simulink model "GCI_Ctrl_PLL_C2000"  (R2024a)
settings: Solver=FixedStepDiscrete  StartTime=0.0  StopTime=8  FixedStep=Sim.ContSampleTime  RelTol=1e-3  EnableMultiTasking=on
values from neighbouring files (symbols this model uses):
  ADPTV = 1.3912    [ModelDD.sldd]
  Ctrl = 0    [ModelDD.sldd]
  EnableMonitors = 0    [ModelDD.sldd]
  FrcPwr = 1    [ModelDD.sldd]
  IdSp = 0.0    [ModelDD.sldd]
  IqSp = 0.0    [ModelDD.sldd]
  ModReq = 1    [ModelDD.sldd]
  PorISel = 0    [ModelDD.sldd]
  PSp = 0.0    [ModelDD.sldd]
  QSp = 0.0    [ModelDD.sldd]
  Sim : value not decoded    [ModelDD.sldd]
  Test = 0    [ModelDD.sldd]
  Var = 650.0    [ModelDD.sldd]
undefined symbols (not defined in the file or in its folder): DiscIntNeverNeededParam, Down, GPTRIP1SEL, GPTRIP2SEL, magnitude, P, TZ1, TZ2, Up
libraries: simulink x38, c2837xDlib x22, c2802xlib x15, slpidlib x9, spsMeanLib x9, spsCurrentMeasurementLib x7, spsThreePhaseVIMeasurementLib x5, spsVoltageMeasurementLib x5, spsTHDLib x4, spsSeriesRLCBranchLib x4, svdutilitieslib x3, c280xlib x3
(part 7 of 11)

== system GCI_Ctrl_PLL_C2000/C2000_SW/CtrlLoop/PLL_Vref/Subsystem/LPF2 ==
  u : Inport
  Alpha : Gain  Gain=(2-w*Ts)/(2+w*Ts)
  Beta : Gain  Gain=(w*Ts)/(2+w*Ts)
  Delay1 : Delay  DelayLength=1  InitialCondition=y_0
  Delay2 : Delay  DelayLength=1
  Sum1 : Sum  Inputs=++|
  Sum2 : Sum  Inputs=|++
  y : Outport  VectorParamsAs1DForOutWhenUnconnected=off
  wires:
  Sum2/1 -> y/1, Delay1/1
  Beta/1 -> Sum2/1
  Sum1/1 -> Beta/1
  Delay2/1 -> Sum1/2
  Alpha/1 -> Sum2/2
  Delay1/1 -> Alpha/1  "y(n-1)"
  u/1 -> Delay2/1, Sum1/1

== system GCI_Ctrl_PLL_C2000/C2000_SW/CtrlLoop/PLL_Vref/Subsystem/PowerCalculation ==
  VdqP : Inport
  VdqN : Inport  Port=2
  IdqzP : Inport  Port=3
  IdqzN : Inport  Port=4
  Add : Sum  Inputs=-+
  Add3 : Sum
  Add4 : Sum
  Demux : Demux  Outputs=2
  Gain4 : Gain  Gain=1.5  ParamDataTypeStr=single
  Gain5 : Gain  Gain=1.5  ParamDataTypeStr=single
  Product{4..7} (4 alike) : Product
  Selector2 : Selector  InputPortWidth=2  IndexOptions=Index vector (dialog)  Indices=[2 1]  OutputSizes=1
  Selector3 : Selector  InputPortWidth=2  IndexOptions=Index vector (dialog)  Indices=[2 1]  OutputSizes=1
  Sum of Elements3 : Sum  Inputs=+
  P0 : Outport  VectorParamsAs1DForOutWhenUnconnected=off
  Q0 : Outport  Port=2  VectorParamsAs1DForOutWhenUnconnected=off
  wires:
  IdqzP/1 -> [IdqP], Selector2/1
  VdqN/1 -> [VdqN]
  IdqzN/1 -> [IdqN], Selector3/1
  VdqP/1 -> [VdqP]
  Product5/1 -> Add3/2
  Add3/1 -> Demux/1
  Product4/1 -> Add3/1
  Add/1 -> Gain4/1
  Gain4/1 -> Q0/1
  Selector2/1 -> [IqdP]
  Selector3/1 -> [IqdN]
  [IqdP] -> Product4/2
  [VdqP] -> Product4/1
  [IqdN] -> Product5/2
  [VdqN] -> Product5/1
  [VdqN] -> Product7/1
  [IdqN] -> Product7/2
  [VdqP] -> Product6/1
  [IdqP] -> Product6/2
  Gain5/1 -> P0/1
  Sum of Elements3/1 -> Gain5/1
  Product6/1 -> Add4/1
  Add4/1 -> Sum of Elements3/1
  Product7/1 -> Add4/2
  Demux/1 -> Add/1
  Demux/2 -> Add/2

== system GCI_Ctrl_PLL_C2000/C2000_SW/CtrlLoop/PLL_Vref/Subsystem/abc_dqz ==
  abc : Inport
  wtNow : Inport  Port=2
  Subsystem : Subsystem
  Subsystem2 : Subsystem
  dqz : Outport  VectorParamsAs1DForOutWhenUnconnected=off
  wires:
  wtNow/1 -> Subsystem2/2(Ang)
  abc/1 -> Subsystem/1(abc)
  Subsystem/1(al_be_0) -> Subsystem2/1(alpha_beta)
  Subsystem2/1(dq) -> dqz/1

== system GCI_Ctrl_PLL_C2000/C2000_SW/CtrlLoop/PLL_Vref/Subsystem/dd_dqz1 ==
  abc : Inport
  wtNow : Inport  Port=2
  Delay : Delay  DelayLength=1
  Delay1 : Delay  DelayLength=1
  Gain : Gain  Gain=-1  ParamDataTypeStr=single
  LPF : Subsystem  mask{Ts=1/(Var.PWM_Freq), w=single(2*pi*50), K=single(1), y_0=0}
      mask prompts: Ts "Sample Time (s)"; w "CutOff Freq (-3db) (rad/s)"; K "Gain"; y_0 "Initial output"
  LPF1 : Subsystem  mask{Ts=1/(Var.PWM_Freq), w=single(2*pi*50), K=single(1), y_0=0}
      mask prompts: Ts "Sample Time (s)"; w "CutOff Freq (-3db) (rad/s)"; K "Gain"; y_0 "Initial output"
  Subsystem : Subsystem
  Subsystem1 : Subsystem
  Subsystem2 : Subsystem
  Subsystem3 : Subsystem
  Subsystem4 : Subsystem
  dqzP : Outport  VectorParamsAs1DForOutWhenUnconnected=off
  dqzN : Outport  Port=2  VectorParamsAs1DForOutWhenUnconnected=off
  wires:
  Subsystem1/1(dq) -> Subsystem3/1(Vdq_in)
  Subsystem2/1(dq) -> Subsystem4/1(Vdq_in)
  Subsystem4/1(Vdq_out) -> LPF/1(u), dqzP/1
  Delay/1 -> Subsystem3/2(Vdq_Inverse)
  Delay1/1 -> Subsystem4/2(Vdq_Inverse)
  Subsystem3/1(Vdq_out) -> LPF1/1(u), dqzN/1
  LPF1/1(y) -> Delay1/1
  LPF/1(y) -> Delay/1
  Gain/1 -> Subsystem1/2(wtNow), Subsystem3/3(Theta)
  abc/1 -> Subsystem/1(abc)
  Subsystem/1(al_be_0) -> Subsystem2/1(alpha_beta), Subsystem1/1(alpha_beta)
  wtNow/1 -> Gain/1, Subsystem2/2(wtNow), Subsystem4/3(Theta)

== system GCI_Ctrl_PLL_C2000/C2000_SW/CtrlLoop/PLL_Vref/Subsystem/dd_dqz2 ==
  abc : Inport
  wtNow : Inport  Port=2
  Delay : Delay  DelayLength=1
  Delay1 : Delay  DelayLength=1
  Gain : Gain  Gain=-1  ParamDataTypeStr=single
  LPF : Subsystem  mask{Ts=1/(Var.PWM_Freq), w=single(50), K=single(1), y_0=0}
      mask prompts: Ts "Sample Time (s)"; w "CutOff Freq (-3db) (rad/s)"; K "Gain"; y_0 "Initial output"
  LPF1 : Subsystem  mask{Ts=1/(Var.PWM_Freq), w=single(50), K=single(1), y_0=0}
      mask prompts: Ts "Sample Time (s)"; w "CutOff Freq (-3db) (rad/s)"; K "Gain"; y_0 "Initial output"
  Subsystem : Subsystem
  Subsystem1 : Subsystem
  Subsystem2 : Subsystem
  Subsystem3 : Subsystem
  Subsystem4 : Subsystem
  dqzP : Outport  VectorParamsAs1DForOutWhenUnconnected=off
  dqzN : Outport  Port=2  VectorParamsAs1DForOutWhenUnconnected=off
  wires:
  Subsystem/1(al_be_0) -> Subsystem1/1(alpha_beta), Subsystem2/1(alpha_beta)
  abc/1 -> Subsystem/1(abc)
  Gain/1 -> Subsystem3/3(Theta), Subsystem1/2(wtNow)
  LPF/1(y) -> Delay/1
  LPF1/1(y) -> Delay1/1
  Subsystem3/1(Vdq_out) -> LPF1/1(u), dqzN/1
  Delay1/1 -> Subsystem4/2(Vdq_Inverse)
  Delay/1 -> Subsystem3/2(Vdq_Inverse)
  Subsystem4/1(Vdq_out) -> LPF/1(u), dqzP/1
  Subsystem2/1(dq) -> Subsystem4/1(Vdq_in)
  Subsystem1/1(dq) -> Subsystem3/1(Vdq_in)
  wtNow/1 -> Gain/1, Subsystem4/3(Theta), Subsystem2/2(wtNow)

== system GCI_Ctrl_PLL_C2000/C2000_SW/CtrlLoop/PLL_Vref/abc2dqzFilt/Single_SOGI ==
  abc : Inport
  Ang : Inport  Port=2
  w : Inport  Port=3
  Subsystem1 : Subsystem
  Subsystem2 : Subsystem
  Subsystem3 : Subsystem
  Dqz : Outport  VectorParamsAs1DForOutWhenUnconnected=off
  dqz_Pll : Outport  Port=2  VectorParamsAs1DForOutWhenUnconnected=off
  wires:
  Subsystem3/1(dq) -> Dqz/1
  Subsystem1/1(AlphBetaCor) -> Subsystem3/1(alpha_beta), Subsystem2/1(alpha_beta)
  w/1 -> Subsystem1/2(w)
  abc/1 -> Subsystem1/1(AlphBeta)
  Ang/1 -> Subsystem2/2(Ang), Subsystem3/2(Ang)
  Subsystem2/1(dq) -> dqz_Pll/1

== system GCI_Ctrl_PLL_C2000/C2000_SW/CtrlLoop/PLL_Vref/abc2dqzFilt/dd_dqz ==
  abc : Inport
  Ang : Inport  Port=2
  w : Inport  Port=3
  Delay : Delay  DelayLength=1
  Delay1 : Delay  DelayLength=1
  Discrete Transfer Fcn3 : DiscreteTransferFcn  Commented=on  Numerator=Var.Filt.Hundms.num  Denominator=Var.Filt.Hundms.den
  Gain : Gain  Gain=-1  ParamDataTypeStr=single
  LPF1 : Subsystem  mask{Ts=1/(Var.PWM_Freq), w=single(50), K=single(1), y_0=0}
      mask prompts: Ts "Sample Time (s)"; w "CutOff Freq (-3db) (rad/s)"; K "Gain"; y_0 "Initial output"
  LPF2 : Subsystem  mask{Ts=1/(Var.PWM_Freq), w=single(50), K=single(1), y_0=0}
      mask prompts: Ts "Sample Time (s)"; w "CutOff Freq (-3db) (rad/s)"; K "Gain"; y_0 "Initial output"
  Subsystem : Subsystem
  Subsystem1 : Subsystem
  Subsystem2 : Subsystem
  Subsystem3 : Subsystem
  Subsystem4 : Subsystem
  Terminator : Terminator
  Dqz : Outport  VectorParamsAs1DForOutWhenUnconnected=off
  dqz_Pll : Outport  Port=2  VectorParamsAs1DForOutWhenUnconnected=off
  wires:
  w/1 -> Terminator/1
  Subsystem/1(al_be_0) -> Subsystem1/1(alpha_beta), Subsystem2/1(alpha_beta)
  abc/1 -> Subsystem/1(abc)
  Ang/1 -> Gain/1, Subsystem4/3(Theta), Subsystem2/2(Ang)
  Gain/1 -> Subsystem3/3(Theta), Subsystem1/2(Ang)
  LPF2/1(y) -> Delay/1
  LPF1/1(y) -> Delay1/1
  Subsystem3/1(Vdq_out) -> LPF1/1(u)
  Delay1/1 -> Subsystem4/2(Vdq_Inverse)
  Delay/1 -> Subsystem3/2(Vdq_Inverse)
  Subsystem4/1(Vdq_out) -> LPF2/1(u), dqz_Pll/1
  Subsystem2/1(dq) -> Subsystem4/1(Vdq_in), Dqz/1
  Subsystem1/1(dq) -> Subsystem3/1(Vdq_in)

== system GCI_Ctrl_PLL_C2000/C2000_SW/CtrlLoop/PLL_Vref/abc2dqzFilt/dd_dqz_SOGI ==
  abc : Inport
  Ang : Inport  Port=2
  w : Inport  Port=3
  Delay : Delay  DelayLength=1
  Delay1 : Delay  DelayLength=1
  Discrete Transfer Fcn1 : DiscreteTransferFcn  Numerator=Var.Filt.Hundms.num  Denominator=Var.Filt.Hundms.den
  Discrete Transfer Fcn2 : DiscreteTransferFcn  Numerator=Var.Filt.Hundms.num  Denominator=Var.Filt.Hundms.den
  Gain : Gain  Gain=-1  ParamDataTypeStr=single
  Subsystem : Subsystem
  Subsystem1 : Subsystem
  Subsystem2 : Subsystem
  Subsystem3 : Subsystem
  Subsystem4 : Subsystem
  Subsystem5 : Subsystem
  dqz_SOGI : Subsystem  VariantControl=Var.Pll.SOGISel == 4
  Dqz : Outport  VectorParamsAs1DForOutWhenUnconnected=off
  dqz_Pll : Outport  Port=2  VectorParamsAs1DForOutWhenUnconnected=off
  wires:
  Delay/1 -> Subsystem3/2(Vdq_Inverse)
  Subsystem2/1(dq) -> Subsystem4/1(Vdq_in), Dqz/1
  abc/1 -> Subsystem/1(abc)
  Delay1/1 -> Subsystem4/2(Vdq_Inverse)
  Subsystem4/1(Vdq_out) -> dqz_Pll/1, Discrete Transfer Fcn1/1
  Discrete Transfer Fcn1/1 -> Delay/1
  Subsystem1/1(dq) -> Subsystem3/1(Vdq_in)
  Subsystem/1(al_be_0) -> Subsystem1/1(alpha_beta), Subsystem2/1(alpha_beta)
  Gain/1 -> Subsystem3/3(Theta), Subsystem1/2(Ang)
  w/1 -> Subsystem5/2(w)
  Ang/1 -> Gain/1, Subsystem4/3(Theta), Subsystem2/2(Ang)
  Subsystem3/1(Vdq_out) -> Discrete Transfer Fcn2/1
  Discrete Transfer Fcn2/1 -> Delay1/1

== system GCI_Ctrl_PLL_C2000/C2000_SW/CtrlLoop/PLL_Vref/abc2dqzFilt/dqz ==
  abc : Inport
  Ang : Inport  Port=2
  w : Inport  Port=3
  Subsystem : Subsystem
  Subsystem2 : Subsystem
  Terminator : Terminator
  Dqz : Outport  VectorParamsAs1DForOutWhenUnconnected=off
  dqz_Pll : Outport  Port=2  VectorParamsAs1DForOutWhenUnconnected=off
  wires:
  abc/1 -> Subsystem/1(abc)
  Subsystem/1(al_be_0) -> Subsystem2/1(alpha_beta)
  Ang/1 -> Subsystem2/2(Ang)
  Subsystem2/1(dq) -> dqz_Pll/1, Dqz/1
  w/1 -> Terminator/1

== system GCI_Ctrl_PLL_C2000/C2000_SW/CtrlLoop/PLL_Vref/abc2dqzFilt/dqz_1P_SOGI_Disc ==
  abc : Inport
  Ang : Inport  Port=2
  w : Inport  Port=3
  SOGI : Subsystem
  Subsystem2 : Subsystem
  Dqz : Outport  VectorParamsAs1DForOutWhenUnconnected=off
  dqz_Pll : Outport  Port=2  VectorParamsAs1DForOutWhenUnconnected=off
  wires:
  Ang/1 -> Subsystem2/2(Ang)
  abc/1 -> SOGI/1(abc)
  w/1 -> SOGI/2(w)
  SOGI/1(AlphBetaCor) -> Subsystem2/1(alpha_beta)
  Subsystem2/1(dq) -> Dqz/1, dqz_Pll/1

== system GCI_Ctrl_PLL_C2000/C2000_SW/CtrlLoop/PLL_Vref/abc2dqzFilt/dqz_DSOGI ==
  abc : Inport
  Ang : Inport  Port=2
  w : Inport  Port=3
  SOGI : Subsystem
  Subsystem : Subsystem
  Subsystem2 : Subsystem
  Subsystem3 : Subsystem
  Dqz : Outport  VectorParamsAs1DForOutWhenUnconnected=off
  dqz_Pll : Outport  Port=2  VectorParamsAs1DForOutWhenUnconnected=off
  wires:
  Subsystem3/1(dq) -> Dqz/1
  SOGI/1(AlphBetaCor) -> Subsystem2/1(alpha_beta)
  w/1 -> SOGI/2(w)
  Subsystem/1(al_be_0) -> SOGI/1(AlphBeta), Subsystem3/1(alpha_beta)
  abc/1 -> Subsystem/1(abc)
  Ang/1 -> Subsystem2/2(Ang), Subsystem3/2(Ang)
  Subsystem2/1(dq) -> dqz_Pll/1

== system GCI_Ctrl_PLL_C2000/C2000_SW/CtrlLoop/PLL_Vref/abc2dqzFilt/dqz_SOGI ==
  abc : Inport
  Ang : Inport  Port=2
  w : Inport  Port=3
  SOGI : Subsystem
  Subsystem : Subsystem
  Subsystem2 : Subsystem
  Subsystem3 : Subsystem
  Dqz : Outport  VectorParamsAs1DForOutWhenUnconnected=off
  dqz_Pll : Outport  Port=2  VectorParamsAs1DForOutWhenUnconnected=off
  wires:
  Subsystem2/1(dq) -> dqz_Pll/1
  Ang/1 -> Subsystem3/2(Ang), Subsystem2/2(Ang)
  abc/1 -> Subsystem/1(abc)
  Subsystem/1(al_be_0) -> Subsystem3/1(alpha_beta), SOGI/1(AlphBeta)
  w/1 -> SOGI/2(w)
  SOGI/1(AlphBetaCor) -> Subsystem2/1(alpha_beta)
  Subsystem3/1(dq) -> Dqz/1

== system GCI_Ctrl_PLL_C2000/C2000_SW/CtrlLoop/PLL_Vref/abc2dqzFilt/dqz_SOGI_ConstW ==
  abc : Inport
  Ang : Inport  Port=2
  w : Inport  Port=3
  Subsystem : Subsystem
  Subsystem1 : Subsystem
  Subsystem2 : Subsystem
  Subsystem3 : Subsystem
  Dqz : Outport  VectorParamsAs1DForOutWhenUnconnected=off
  dqz_Pll : Outport  Port=2  VectorParamsAs1DForOutWhenUnconnected=off
  wires:
  Subsystem3/1(dq) -> Dqz/1
  Subsystem1/1(AlphBetaCor) -> Subsystem2/1(alpha_beta)
  w/1 -> Subsystem1/2(w)
  Subsystem/1(al_be_0) -> Subsystem1/1(AlphBeta), Subsystem3/1(alpha_beta)
  abc/1 -> Subsystem/1(abc)
  Ang/1 -> Subsystem2/2(Ang), Subsystem3/2(Ang)
  Subsystem2/1(dq) -> dqz_Pll/1

== system GCI_Ctrl_PLL_C2000/C2000_SW/CtrlLoop/PLL_Vref/abc2dqzFilt/dqz_SOGI_Disc ==
  abc : Inport
  Ang : Inport  Port=2
  w : Inport  Port=3
  SOGI : Subsystem
  Subsystem : Subsystem
  Subsystem2 : Subsystem
  Subsystem3 : Subsystem
  Dqz : Outport  VectorParamsAs1DForOutWhenUnconnected=off
  dqz_Pll : Outport  Port=2  VectorParamsAs1DForOutWhenUnconnected=off
  wires:
  Subsystem3/1(dq) -> Dqz/1
  SOGI/1(AlphBetaCor) -> Subsystem2/1(alpha_beta)
  w/1 -> SOGI/2(w)
  Subsystem/1(al_be_0) -> SOGI/1(AlphBeta), Subsystem3/1(alpha_beta)
  abc/1 -> Subsystem/1(abc)
  Ang/1 -> Subsystem2/2(Ang), Subsystem3/2(Ang)
  Subsystem2/1(dq) -> dqz_Pll/1

== system GCI_Ctrl_PLL_C2000/C2000_SW/CtrlLoop/ADC Scaling/ADC Scaling 3 Cur/RemoveDCOffset/LPF ==
  VabcGrid : Inport
  Rst : Inport  Port=2
  LPF1 : Subsystem  mask{Ts=1/(Var.PWM_Freq), w=single(2*pi*0.1), K=single(1), y_0=0}
      mask prompts: Ts "Sample Time (s)"; w "CutOff Freq (-3db) (rad/s)"; K "Gain"; y_0 "Initial output"
  Saturation : Saturate  UpperLimit=50  LowerLimit=-50
  Subtract : Sum  Inputs=+-
  VabcGridAdj : Outport  VectorParamsAs1DForOutWhenUnconnected=off
  VabcGridOff : Outport  Port=2  VectorParamsAs1DForOutWhenUnconnected=off
  wires:
  Saturation/1 -> Subtract/2, VabcGridOff/1
  Subtract/1 -> VabcGridAdj/1  "VgabcAdj"
  VabcGrid/1 -> LPF1/1(VabcGrid), Subtract/1
  LPF1/1(y) -> Saturation/1
  Rst/1 -> LPF1/2(rst)

== system GCI_Ctrl_PLL_C2000/C2000_SW/CtrlLoop/ADC Scaling/ADC Scaling 3 Cur/RemoveDCOffset/None ==
  VabcGrid : Inport
  VabcGridAdj : Outport  VectorParamsAs1DForOutWhenUnconnected=off
  wires:
  VabcGrid/1 -> VabcGridAdj/1

== system GCI_Ctrl_PLL_C2000/C2000_SW/CtrlLoop/ADC Scaling/ADC Scaling 3 Cur/Subsystem/LPF ==
  VabcGrid : Inport
  Alpha : Gain  Gain=(2-w*Ts)/(2+w*Ts)
  Beta : Gain  Gain=(w*Ts)/(2+w*Ts)
  Delay1 : Delay  DelayLength=1  InitialCondition=y_0
  Delay2 : Delay  DelayLength=1
  Sum1 : Sum  Inputs=++|
  Sum2 : Sum  Inputs=|++
  y : Outport  Unit=A  VectorParamsAs1DForOutWhenUnconnected=off
  wires:
  Sum2/1 -> y/1, Delay1/1  "VgabcDcOffFil"
  Beta/1 -> Sum2/1
  Sum1/1 -> Beta/1
  Delay2/1 -> Sum1/2
  Alpha/1 -> Sum2/2
  Delay1/1 -> Alpha/1  "y(n-1)"
  VabcGrid/1 -> Delay2/1, Sum1/1

== system GCI_Ctrl_PLL_C2000/C2000_SW/CtrlLoop/ADC Scaling/ADC Scaling 3 Volts/RemoveDCOffset/LPF ==
  VabcGrid : Inport
  LPF : Subsystem  mask{Ts=1/(Var.PWM_Freq), w=single(2*pi*0.1), K=single(1), y_0=0}
      mask prompts: Ts "Sample Time (s)"; w "CutOff Freq (-3db) (rad/s)"; K "Gain"; y_0 "Initial output"
  Saturation : Saturate  UpperLimit=50  LowerLimit=-50
  Subtract : Sum  Inputs=+-
  VabcGridAdj : Outport  VectorParamsAs1DForOutWhenUnconnected=off
  VabcGridOff : Outport  Port=2  VectorParamsAs1DForOutWhenUnconnected=off
  wires:
  LPF/1(y) -> Saturation/1
  VabcGrid/1 -> LPF/1(VabcGrid), Subtract/1
  Subtract/1 -> VabcGridAdj/1  "VgabcAdj"
  Saturation/1 -> VabcGridOff/1, Subtract/2

== system GCI_Ctrl_PLL_C2000/C2000_SW/CtrlLoop/ADC Scaling/ADC Scaling 3 Volts/RemoveDCOffset/None ==
  VabcGrid : Inport
  VabcGridAdj : Outport  VectorParamsAs1DForOutWhenUnconnected=off
  wires:
  VabcGrid/1 -> VabcGridAdj/1

== system GCI_Ctrl_PLL_C2000/C2000_SW/CtrlLoop/ADC Scaling/ADC Scaling 3 Volts/Subsystem/LPF ==
  VabcGrid : Inport
  Alpha : Gain  Gain=(2-w*Ts)/(2+w*Ts)
  Beta : Gain  Gain=(w*Ts)/(2+w*Ts)
  Delay1 : Delay  DelayLength=1  InitialCondition=y_0
  Delay2 : Delay  DelayLength=1
  Sum1 : Sum  Inputs=++|
  Sum2 : Sum  Inputs=|++
  y : Outport  VectorParamsAs1DForOutWhenUnconnected=off
  wires:
  VabcGrid/1 -> Sum1/1, Delay2/1
  Delay1/1 -> Alpha/1  "y(n-1)"
  Alpha/1 -> Sum2/2
  Delay2/1 -> Sum1/2
  Sum1/1 -> Beta/1
  Beta/1 -> Sum2/1
  Sum2/1 -> Delay1/1, y/1  "VgabcDcOffFil"

== system GCI_Ctrl_PLL_C2000/C2000_SW/CtrlLoop/CurrentController/CurrentController/Subsystem/PowerCalculation ==
  VdqP : Inport
  VdqN : Inport  Port=2
  IdqzP : Inport  Port=3
  IdqzN : Inport  Port=4
  Add : Sum  Inputs=-+
  Add3 : Sum
  Add4 : Sum
  Demux : Demux  Outputs=2
  Gain4 : Gain  Gain=1.5  ParamDataTypeStr=single
  Gain5 : Gain  Gain=1.5  ParamDataTypeStr=single
  Product{4..7} (4 alike) : Product
  Selector2 : Selector  InputPortWidth=2  IndexOptions=Index vector (dialog)  Indices=[2 1]  OutputSizes=1
  Selector3 : Selector  InputPortWidth=2  IndexOptions=Index vector (dialog)  Indices=[2 1]  OutputSizes=1
  Sum of Elements3 : Sum  Inputs=+
  P0 : Outport  VectorParamsAs1DForOutWhenUnconnected=off
  Q0 : Outport  Port=2  VectorParamsAs1DForOutWhenUnconnected=off
  wires:
  IdqzP/1 -> [IdqP], Selector2/1
  VdqN/1 -> [VdqN]
  IdqzN/1 -> [IdqN], Selector3/1
  VdqP/1 -> [VdqP]
  Product5/1 -> Add3/2
  Add3/1 -> Demux/1
  Product4/1 -> Add3/1
  Add/1 -> Gain4/1
  Gain4/1 -> Q0/1
  Selector2/1 -> [IqdP]
  Selector3/1 -> [IqdN]
  [IqdP] -> Product4/2
  [VdqP] -> Product4/1
  [IqdN] -> Product5/2
  [VdqN] -> Product5/1
  [VdqN] -> Product7/1
  [IdqN] -> Product7/2
  [VdqP] -> Product6/1
  [IdqP] -> Product6/2
  Gain5/1 -> P0/1
  Sum of Elements3/1 -> Gain5/1
  Product6/1 -> Add4/1
  Add4/1 -> Sum of Elements3/1
  Product7/1 -> Add4/2
  Demux/1 -> Add/1
  Demux/2 -> Add/2

== system GCI_Ctrl_PLL_C2000/C2000_SW/CtrlLoop/CurrentController/CurrentController/Subsystem/abc_dqz ==
  abc : Inport
  wtNow : Inport  Port=2
  Subsystem : Subsystem
  Subsystem2 : Subsystem
  dqz : Outport  VectorParamsAs1DForOutWhenUnconnected=off
  wires:
  wtNow/1 -> Subsystem2/2(Ang)
  abc/1 -> Subsystem/1(abc)
  Subsystem/1(al_be_0) -> Subsystem2/1(alpha_beta)
  Subsystem2/1(dq) -> dqz/1

== system GCI_Ctrl_PLL_C2000/C2000_SW/CtrlLoop/CurrentController/CurrentController/Subsystem/dd_dqz1 ==
  abc : Inport
  wtNow : Inport  Port=2
  Delay : Delay  DelayLength=1
  Delay1 : Delay  DelayLength=1
  Gain : Gain  Gain=-1  ParamDataTypeStr=single
  LPF : Subsystem  mask{Ts=1/(Var.PWM_Freq), w=single(2*pi*50), K=single(1), y_0=0}
      mask prompts: Ts "Sample Time (s)"; w "CutOff Freq (-3db) (rad/s)"; K "Gain"; y_0 "Initial output"
  LPF1 : Subsystem  mask{Ts=1/(Var.PWM_Freq), w=single(2*pi*50), K=single(1), y_0=0}
      mask prompts: Ts "Sample Time (s)"; w "CutOff Freq (-3db) (rad/s)"; K "Gain"; y_0 "Initial output"
  Subsystem : Subsystem
  Subsystem1 : Subsystem
  Subsystem2 : Subsystem
  Subsystem3 : Subsystem
  Subsystem4 : Subsystem
  dqzP : Outport  VectorParamsAs1DForOutWhenUnconnected=off
  dqzN : Outport  Port=2  VectorParamsAs1DForOutWhenUnconnected=off
  wires:
  Subsystem1/1(dq) -> Subsystem3/1(Vdq_in)
  Subsystem2/1(dq) -> Subsystem4/1(Vdq_in)
  Subsystem4/1(Vdq_out) -> LPF/1(u), dqzP/1
  Delay/1 -> Subsystem3/2(Vdq_Inverse)
  Delay1/1 -> Subsystem4/2(Vdq_Inverse)
  Subsystem3/1(Vdq_out) -> LPF1/1(u), dqzN/1
  LPF1/1(y) -> Delay1/1
  LPF/1(y) -> Delay/1
  Gain/1 -> Subsystem1/2(wtNow), Subsystem3/3(Theta)
  abc/1 -> Subsystem/1(abc)
  Subsystem/1(al_be_0) -> Subsystem2/1(alpha_beta), Subsystem1/1(alpha_beta)
  wtNow/1 -> Gain/1, Subsystem2/2(wtNow), Subsystem4/3(Theta)

== system GCI_Ctrl_PLL_C2000/C2000_SW/CtrlLoop/CurrentController/CurrentController/Subsystem/dd_dqz2 ==
  abc : Inport
  wtNow : Inport  Port=2
  Delay : Delay  DelayLength=1
  Delay1 : Delay  DelayLength=1
  Gain : Gain  Gain=-1  ParamDataTypeStr=single
  LPF : Subsystem  mask{Ts=1/(Var.PWM_Freq), w=single(50), K=single(1), y_0=0}
      mask prompts: Ts "Sample Time (s)"; w "CutOff Freq (-3db) (rad/s)"; K "Gain"; y_0 "Initial output"
  LPF1 : Subsystem  mask{Ts=1/(Var.PWM_Freq), w=single(50), K=single(1), y_0=0}
      mask prompts: Ts "Sample Time (s)"; w "CutOff Freq (-3db) (rad/s)"; K "Gain"; y_0 "Initial output"
  Subsystem : Subsystem
  Subsystem1 : Subsystem
  Subsystem2 : Subsystem
  Subsystem3 : Subsystem
  Subsystem4 : Subsystem
  dqzP : Outport  VectorParamsAs1DForOutWhenUnconnected=off
  dqzN : Outport  Port=2  VectorParamsAs1DForOutWhenUnconnected=off
  wires:
  Subsystem/1(al_be_0) -> Subsystem1/1(alpha_beta), Subsystem2/1(alpha_beta)
  abc/1 -> Subsystem/1(abc)
  Gain/1 -> Subsystem3/3(Theta), Subsystem1/2(wtNow)
  LPF/1(y) -> Delay/1
  LPF1/1(y) -> Delay1/1
  Subsystem3/1(Vdq_out) -> LPF1/1(u), dqzN/1
  Delay1/1 -> Subsystem4/2(Vdq_Inverse)
  Delay/1 -> Subsystem3/2(Vdq_Inverse)
  Subsystem4/1(Vdq_out) -> LPF/1(u), dqzP/1
  Subsystem2/1(dq) -> Subsystem4/1(Vdq_in)
  Subsystem1/1(dq) -> Subsystem3/1(Vdq_in)
  wtNow/1 -> Gain/1, Subsystem4/3(Theta), Subsystem2/2(wtNow)

== system GCI_Ctrl_PLL_C2000/C2000_SW/CtrlLoop/CurrentController/CurrentController/dqz2abc_1/Subsystem ==
  al_be_0 : Inport  OutDataTypeStr=single  PortDimensions=3
  Gain3 : Gain  Gain="single([ 1   0   1; -1/2  sqrt(3)/2   1; -1/2  -sqrt(3)/2  1 ] )"  Multiplication=Matrix(K*u) (u vector)  ParamDataTypeStr=single  OutDataTypeStr=single  SaturateOnIntegerOverflow=on
  abc : Outport  OutDataTypeStr=single  VectorParamsAs1DForOutWhenUnconnected=off
  wires:
  al_be_0/1 -> Gain3/1
  Gain3/1 -> abc/1  "abc"

== system GCI_Ctrl_PLL_C2000/C2000_SW/CtrlLoop/CurrentController/CurrentController/dqz2abc_1/Subsystem1 ==
  note: =
  note: =
  note: *
  note: [ d
      |    q ]
  note: [  al
      |     be  ]
  note: [ d
      |    q ]
  note: inv ([  cos(wt)   sin(wt)
      |    -sin(wt)    cos(wt)   ])
  note: [  al
      |     be  ]
  note: [  cos(wt)   -sin(wt)
      |    sin(wt)    cos(wt)   ]
  note: *
  dqz : Inport  OutDataTypeStr=single  PortDimensions=3
  Ang : Inport  Port=2  OutDataTypeStr=single  PortDimensions=1
  Fcn : Fcn  Expr=u[1]*cos(u[3]) - u[2]*sin(u[3])
  Fcn1 : Fcn  Expr=u[1]*sin(u[3]) + u[2]*cos(u[3])
  Mux1 : Mux  Inputs=3
  Mux2 : Mux  Inputs=[2 1]
  Mux3 : Mux  Inputs=[2 1]
  Selector : Selector  InputPortWidth=3  IndexOptions=Index vector (dialog)  Indices=[1 2]  OutputSizes=1
  Selector1 : Selector  InputPortWidth=3  IndexOptions=Index vector (dialog)  Indices=[3]  OutputSizes=1
  alpha_beta : Outport  OutDataTypeStr=single  InitialOutput=[0,0]  VectorParamsAs1DForOutWhenUnconnected=off
  wires:
  Selector1/1 -> Mux1/3
  dqz/1 -> Selector/1, Selector1/1
  Selector/1 -> Mux3/1, Mux2/1
  Fcn/1 -> Mux1/1
  Ang/1 -> Mux3/2, Mux2/2
  Mux2/1 -> Fcn/1
  Mux1/1 -> alpha_beta/1
  Mux3/1 -> Fcn1/1
  Fcn1/1 -> Mux1/2

== system GCI_Ctrl_PLL_C2000/C2000_SW/CtrlLoop/CurrentController/CurrentControllerAdptv/MESO/CFDL ==
  u_k-1 : Inport
  e_k : Inport  Port=2
  Abs : Abs  SaturateOnIntegerOverflow=off
  Compare To Constant : simulink/Logic and Bit Operations/Compare To Constant  relop=>  const=0  OutDataTypeStr=boolean
  Compare To Constant1 : simulink/Logic and Bit Operations/Compare To Constant  relop=>=  const=ADPTV.k*eye(size(ADPTV.psi0,1),size(ADPTV.psi0,2))  OutDataTypeStr=boolean
  Delta : Gain  Gain=ADPTV.delta
  Divide : Product  Inputs=*/
  Mag : Subsystem
  Product : Product  Multiplication=Matrix(*)
  Product1 : Product  Multiplication=Matrix(*)
  Product3 : Product
  Psi_0 : Constant  Value=ADPTV.psi0
  Reshape : Reshape  OutputDimensionality=Column vector (2-D)
  Square : Math  Operator=square
  Sum : Sum  Inputs=|+-
  Sum1 : Sum  Inputs=|+-
  Sum2 : Sum  Inputs=|+-
  Sum3 : Sum  Inputs=|++
  Sum4 : Sum  Inputs=|++
  Switch : Switch  Criteria=u2 > Threshold  SaturateOnIntegerOverflow=off  InputSameDT=off
  Switch1 : Switch  Criteria=u2 > Threshold  SaturateOnIntegerOverflow=off  InputSameDT=off
  Transpose : Math  Operator=transpose
  Unit Delay : UnitDelay  InitialCondition=ADPTV.psi0  SampleTime=-1  HasFrameUpgradeWarning=on
  Unit Delay1 : UnitDelay  SampleTime=-1  HasFrameUpgradeWarning=on
  Unit Delay2 : UnitDelay  SampleTime=-1  HasFrameUpgradeWarning=on
  eta : Constant  Value=ADPTV.eta
  Phi_k : Outport
  wires:
  Sum4/1 -> Product3/1, Switch/1  "Phi_k"
  Unit Delay/1 -> [Phi_k_1]  "$\\hat{\\Phi}_{e,k-1}$"
  u_k-1/1 -> Sum/1, Unit Delay1/1
  Unit Delay1/1 -> Sum/2
  Sum/1 -> [D_u_k_1], Mag/1(In1), Transpose/1  "$\\Delta u_{k-1}$"
  Mag/1(Out1) -> [Abs_D_u_k_1]  "$||\\Delta u_{k-1}||$"
  Transpose/1 -> [D_u_k_1_T]
  Sum1/1 -> [D_e_k]  "$\\Delta e_{k}$"
  Unit Delay2/1 -> Sum1/2
  e_k/1 -> Unit Delay2/1, Sum1/1
  [D_e_k] -> Sum2/1
  Product/1 -> Sum2/2
  [Phi_k_1] -> Product/1
  [D_u_k_1] -> Product/2
  Sum2/1 -> Delta/1
  [D_u_k_1_T] -> Product1/2
  [Abs_D_u_k_1] -> Square/1
  eta/1 -> Sum3/1
  Product1/1 -> Divide/1  "$\\delta(\\Delta e_{k}-\\hat{\\Phi}_{e,k-1}\\Delta u_{k-1})\\Delta u_{k-1}^T$"
  Sum3/1 -> Divide/2  "$\\eta+||\\Delta u_{k-1}||^2$"
  Square/1 -> Sum3/2  "$||\\Delta u_{k-1}||^2$"
  Divide/1 -> Sum4/1  "$\\frac{\\delta(\\Delta e_{k}-\\hat{\\Phi}_{e,k-1}\\Delta u_{k-1})\\Delta u_{k-1}^T}{\\eta+||\\Delta u_{k-1}||^2}$"
  [Phi_k_1] -> Sum4/2
  Psi_0/1 -> Switch/3, Switch1/3, Product3/2
  Compare To Constant/1 -> Switch/2
  Switch/1 -> Abs/1, Switch1/1
  Product3/1 -> Compare To Constant/1
  Abs/1 -> Compare To Constant1/1
  Compare To Constant1/1 -> Switch1/2
  Switch1/1 -> Phi_k/1, Unit Delay/1
  Delta/1 -> Reshape/1
  Reshape/1 -> Product1/1

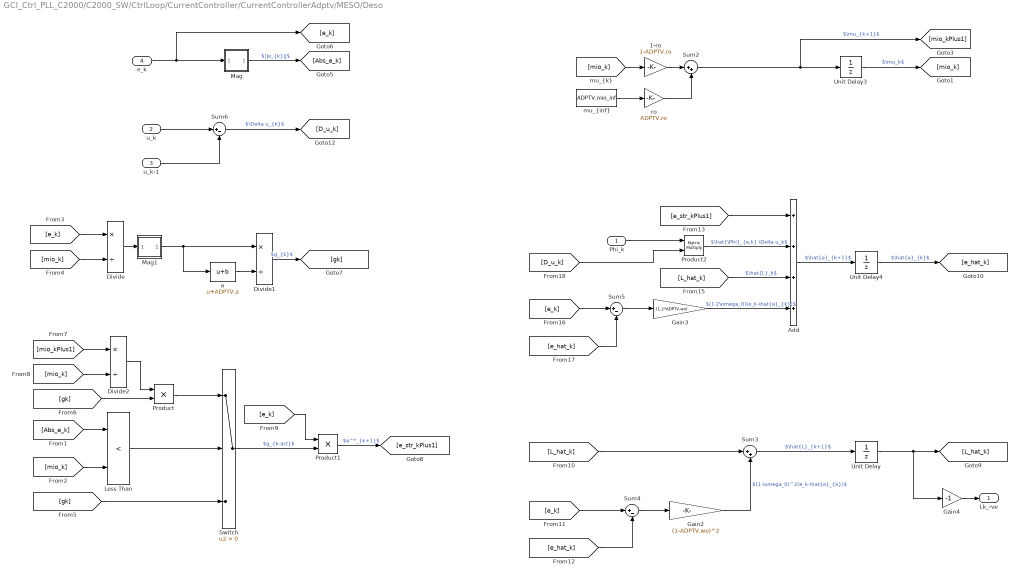
== system GCI_Ctrl_PLL_C2000/C2000_SW/CtrlLoop/CurrentController/CurrentControllerAdptv/MESO/Deso ==
  Phi_k : Inport
  u_k : Inport  Port=2
  u_k-1 : Inport  Port=3
  e_k : Inport  Port=4
  1-ro : Gain  Gain=1-ADPTV.ro
  Add : Sum  Inputs=++++
  Divide : Product  Inputs=*/
  Divide1 : Product  Inputs=*/
  Divide2 : Product  Inputs=*/
  Gain2 : Gain  Gain=(1-ADPTV.wo)^2
  Gain3 : Gain  Gain=(1-2*ADPTV.wo)
  Gain4 : Gain  Gain=-1
  Less Than : RelationalOperator  Operator=<  OutDataTypeStr=boolean  RndMeth=Simplest  InputSameDT=off
  Mag : Subsystem
  Mag1 : Subsystem
  Product : Product
  Product1 : Product
  Product2 : Product  Multiplication=Matrix(*)
  Sum2 : Sum  Inputs=|++
  Sum3 : Sum  Inputs=|++
  Sum4 : Sum  Inputs=|+-
  Sum5 : Sum  Inputs=|+-
  Sum6 : Sum  Inputs=|+-
  Switch : Switch  Criteria=u2 > Threshold  SaturateOnIntegerOverflow=off  InputSameDT=off
  Unit Delay : UnitDelay  SampleTime=-1  HasFrameUpgradeWarning=on
  Unit Delay3 : UnitDelay  InitialCondition=ADPTV.mio_0  SampleTime=-1  HasFrameUpgradeWarning=on
  Unit Delay4 : UnitDelay  SampleTime=-1  HasFrameUpgradeWarning=on
  a : Bias  Bias=ADPTV.a  SaturateOnIntegerOverflow=off
  "mu_{inf}" : Constant  Value=ADPTV.mio_inf
  ro : Gain  Gain=ADPTV.ro
  Lk_-ve : Outport
  wires:
  Unit Delay3/1 -> [mio_k]  "$\\mu_k$"
  Sum2/1 -> [mio_kPlus1], Unit Delay3/1  "$\\mu_{k+1}$"
  "mu_{inf}"/1 -> ro/1
  ro/1 -> Sum2/2
  1-ro/1 -> Sum2/1
  [mio_k] -> 1-ro/1
  e_k/1 -> [e_k], Mag/1(e_k)
  Mag/1(Out1) -> [Abs_e_k]  "$||e_{k}||$"
  [Abs_e_k] -> Less Than/1
  [mio_k] -> Less Than/2
  Less Than/1 -> Switch/2
  [e_k] -> Divide/1
  [mio_k] -> Divide/2
  Divide/1 -> Mag1/1(e_k)
  Mag1/1(Out1) -> Divide1/1, a/1
  a/1 -> Divide1/2
  Divide1/1 -> [gk]  "$g_{k}$"
  [gk] -> Switch/3
  [mio_k] -> Divide2/2
  [mio_kPlus1] -> Divide2/1
  [gk] -> Product/2
  Divide2/1 -> Product/1
  Product/1 -> Switch/1
  Switch/1 -> Product1/2  "$g_{k-act}$"
  [e_k] -> Product1/1
  Product1/1 -> [e_str_kPlus1]  "$e^*_{k+1}$"
  [L_hat_k] -> Sum3/1
  Unit Delay/1 -> Gain4/1, [L_hat_k]
  Sum4/1 -> Gain2/1
  Gain2/1 -> Sum3/2  "$(1-\\omega_0)^2(e_k-\\hat{e}_{k})$"
  [e_k] -> Sum4/1
  [e_hat_k] -> Sum4/2
  Sum3/1 -> Unit Delay/1  "$\\hat{L}_{k+1}$"
  Unit Delay4/1 -> [e_hat_k]  "$\\hat{e}_{k}$"
  Add/1 -> Unit Delay4/1  "$\\hat{e}_{k+1}$"
  Phi_k/1 -> Product2/1
  [D_u_k] -> Product2/2
  [e_str_kPlus1] -> Add/1
  Product2/1 -> Add/2  "$\\hat{\\Phi}_{e,k} \\Delta u_k$"
  [L_hat_k] -> Add/3  "$\\hat{L}_k$"
  [e_hat_k] -> Sum5/2
  [e_k] -> Sum5/1
  Sum5/1 -> Gain3/1
  Gain4/1 -> Lk_-ve/1
  Sum6/1 -> [D_u_k]  "$\\Delta u_{k}$"
  u_k/1 -> Sum6/1
  Gain3/1 -> Add/4  "$(1-2\\omega_0)(e_k-\\hat{e}_{k})$"
  u_k-1/1 -> Sum6/2

== system GCI_Ctrl_PLL_C2000/C2000_SW/CtrlLoop/CurrentController/CurrentControllerAdptv/MESO/Lambda ==
  Bias : Bias  Bias=ADPTV.LamdaInf  SaturateOnIntegerOverflow=off
  Constant2 : Constant  Value=ADPTV.Lamda0-ADPTV.LamdaInf
  Constant3 : Constant
  Data Type Conversion : DataTypeConversion  SaturateOnIntegerOverflow=off  RndMeth=Floor
  Discrete-Time Integrator : DiscreteIntegrator  SampleTime=-1  ICPrevOutput=DiscIntNeverNeededParam  ICPrevScaledInput=DiscIntNeverNeededParam
  Gain : Gain  Gain=-ADPTV.b0
  Math Function1 : Math
  Product3 : Product
  $\lambda_k$ : Outport
  wires:
  Constant2/1 -> Product3/2
  Discrete-Time Integrator/1 -> Gain/1
  Constant3/1 -> Discrete-Time Integrator/1
  Gain/1 -> Math Function1/1
  Math Function1/1 -> Data Type Conversion/1
  Product3/1 -> Bias/1
  Bias/1 -> $\lambda_k$/1  "$\\lambda_k$"
  Data Type Conversion/1 -> Product3/1

== system GCI_Ctrl_PLL_C2000/C2000_SW/CtrlLoop/CurrentController/CurrentControllerAdptv/MESO/Mag ==
  in : Inport
  Reshape : Reshape
  Sqrt : Sqrt
  Square : Math  Operator=square
  Sum of Elements : Sum  Inputs=+
  Abs : Outport
  wires:
  Sqrt/1 -> Reshape/1
  Sum of Elements/1 -> Sqrt/1
  Square/1 -> Sum of Elements/1
  in/1 -> Square/1
  Reshape/1 -> Abs/1

== system GCI_Ctrl_PLL_C2000/C2000_SW/CtrlLoop/CurrentController/CurrentControllerAdptv/MESO/Mag1 ==
  in : Inport
  Gain : Gain  Gain=4
  Gain1 : Gain  Gain=0.5
  Product : Product
  Product1 : Product
  Selector : Selector  NumberOfDimensions=2  InputPortWidth=3  IndexOptions=Index vector (dialog),Index vector (dialog)  Indices=1,1  OutputSizes=1,1
  Selector1 : Selector  NumberOfDimensions=2  InputPortWidth=3  IndexOptions=Index vector (dialog),Index vector (dialog)  Indices=2,2  OutputSizes=1,1
  Selector2 : Selector  NumberOfDimensions=2  InputPortWidth=3  IndexOptions=Index vector (dialog),Index vector (dialog)  Indices=1,2  OutputSizes=1,1
  Selector3 : Selector  NumberOfDimensions=2  InputPortWidth=3  IndexOptions=Index vector (dialog),Index vector (dialog)  Indices=2,1  OutputSizes=1,1
  Sqrt1 : Sqrt
  Sqrt2 : Sqrt
  Square : Math  Operator=square
  Square1 : Math  Operator=square
  Square2 : Math  Operator=square
  Sum : Sum  Inputs=|+-
  Sum of Elements : Sum  Inputs=+
  Sum1 : Sum  Inputs=|+-
  Sum2 : Sum  Inputs=|+-
  Abs : Outport
  wires:
  Square/1 -> Sum of Elements/1
  in/1 -> Selector1/1, Selector2/1, Selector3/1, Selector/1, Square/1
  Sum of Elements/1 -> Sum2/1, Square1/1
  Selector/1 -> Product/1
  Selector1/1 -> Product/2
  Selector3/1 -> Product1/2
  Selector2/1 -> Product1/1
  Product/1 -> Sum/1
  Product1/1 -> Sum/2
  Sum/1 -> [det]
  [det] -> Square2/1
  Square2/1 -> Gain/1
  Square1/1 -> Sum1/1
  Gain/1 -> Sum1/2
  Sum1/1 -> Sqrt1/1
  Sqrt1/1 -> Sum2/2
  Sum2/1 -> Gain1/1
  Gain1/1 -> Sqrt2/1
  Sqrt2/1 -> Abs/1

== system GCI_Ctrl_PLL_C2000/C2000_SW/CtrlLoop/CurrentController/CurrentControllerAdptv/MESO/Mag2 ==
  in : Inport
  Constant : Constant  OutDataTypeStr=single
  Fcn : Fcn  Expr=(u[2]+sqrt(u[2]^2 - 4*u[1]*u[3]))/(2*u[1])
  Fcn1 : Fcn  Expr=(u[2]-sqrt(u[2]^2 - 4*u[1]*u[3]))/(2*u[1])
  Matrix Multiply : Product  Multiplication=Matrix(*)
  Max : MinMax  Function=max  Inputs=2
  Mux : Mux  Inputs=3
  Product : Product
  Product1 : Product
  Reshape{,1..4} (5 alike) : Reshape
  Selector : Selector  NumberOfDimensions=2  InputPortWidth=3  IndexOptions=Index vector (dialog),Index vector (dialog)  Indices=1,1  OutputSizes=1,1
  Selector1 : Selector  NumberOfDimensions=2  InputPortWidth=3  IndexOptions=Index vector (dialog),Index vector (dialog)  Indices=1,2  OutputSizes=1,1
  Selector2 : Selector  NumberOfDimensions=2  InputPortWidth=3  IndexOptions=Index vector (dialog),Index vector (dialog)  Indices=2,1  OutputSizes=1,1
  Selector3 : Selector  NumberOfDimensions=2  InputPortWidth=3  IndexOptions=Index vector (dialog),Index vector (dialog)  Indices=2,2  OutputSizes=1,1
  Sqrt3 : Sqrt
  Sum : Sum  Inputs=|++
  Sum1 : Sum  Inputs=|+-
  Transpose : matrix_library/Transpose
  Abs : Outport
  wires:
  Reshape/1 -> Abs/1
  Transpose/1 -> Matrix Multiply/1
  in/1 -> Matrix Multiply/2, Transpose/1
  Max/1 -> Sqrt3/1
  Sqrt3/1 -> Reshape/1
  Selector/1 -> Reshape1/1
  Reshape1/1 -> Product1/1, Sum/1  "a"
  Selector3/1 -> Reshape4/1
  Selector2/1 -> Reshape3/1
  Selector1/1 -> Reshape2/1
  Reshape2/1 -> Product/1  "b"
  Reshape3/1 -> Product/2  "c"
  Reshape4/1 -> Product1/2, Sum/2  "d"
  Mux/1 -> Fcn1/1, Fcn/1
  Fcn/1 -> Max/1
  Fcn1/1 -> Max/2
  Sum/1 -> Mux/2
  Product/1 -> Sum1/1
  Product1/1 -> Sum1/2
  Sum1/1 -> Mux/3
  Constant/1 -> Mux/1
  Matrix Multiply/1 -> Selector3/1, Selector2/1, Selector1/1, Selector/1

== system GCI_Ctrl_PLL_C2000/C2000_SW/CtrlLoop/CurrentController/CurrentControllerAdptv/MESO/Subsystem ==
  $v_k$ : Inport
  "$u_{k-1}$" : Inport  Port=2
  Abs : Abs  SaturateOnIntegerOverflow=off
  Constant : Constant  Value=ADPTV.b_D_ui
  Constant1 : Constant  Value=ADPTV.b_D_ui
  Less Than : RelationalOperator  Operator=<  OutDataTypeStr=boolean  RndMeth=Simplest  InputSameDT=off
  Product : Product
  Sign : Signum
  Sum6 : Sum  Inputs=|++
  Switch : Switch  Criteria=u2 > Threshold  SaturateOnIntegerOverflow=off  InputSameDT=off
  $u_k$ : Outport
  wires:
  Sign/1 -> Product/1
  [ui_cond] -> Switch/2
  Less Than/1 -> [ui_cond]  "$u_{sat}$"
  $v_k$/1 -> Sign/1, Abs/1, Switch/1
  Constant/1 -> Less Than/2
  Product/1 -> Switch/3
  Constant1/1 -> Product/2
  Abs/1 -> Less Than/1
  Switch/1 -> Sum6/1
  Sum6/1 -> $u_k$/1  "$u_k$"
  "$u_{k-1}$"/1 -> Sum6/2

== system GCI_Ctrl_PLL_C2000/C2000_SW/CtrlLoop/CurrentController/CurrentControllerAdptv/Phase2Line/Line ==
  In : Inport
  Demux : Demux  Outputs=3
  Gain : Gain  Gain=single(1/3)  ParamDataTypeStr=single
  Gain1 : Gain  Gain=single(1/3)  ParamDataTypeStr=single
  Gain2 : Gain  Gain=single(1/3)  ParamDataTypeStr=single
  Mux : Mux  Inputs=3
  Sum : Sum  Inputs=|+-
  Sum1 : Sum  Inputs=-+|
  Sum2 : Sum  Inputs=-+|
  Out : Outport
  wires:
  Mux/1 -> Out/1
  Gain/1 -> Mux/1
  Gain2/1 -> Mux/3
  Gain1/1 -> Mux/2
  Sum1/1 -> Gain1/1
  Sum2/1 -> Gain2/1
  Sum/1 -> Gain/1
  Demux/2 -> Sum1/2, Sum2/1
  Demux/3 -> Sum/2, Sum2/2
  Demux/1 -> Sum/1, Sum1/1
  In/1 -> Demux/1

== system GCI_Ctrl_PLL_C2000/C2000_SW/CtrlLoop/CurrentController/CurrentControllerAdptv/Phase2Line/Phase ==
  In : Inport
  Out : Outport
  wires:
  In/1 -> Out/1

== system GCI_Ctrl_PLL_C2000/C2000_SW/CtrlLoop/CurrentController/CurrentControllerAdptv/Subsystem/PowerCalculation ==
  VdqP : Inport
  VdqN : Inport  Port=2
  IdqzP : Inport  Port=3
  IdqzN : Inport  Port=4
  Add : Sum  Inputs=-+
  Add3 : Sum
  Add4 : Sum
  Demux : Demux  Outputs=2
  Gain4 : Gain  Gain=1.5  ParamDataTypeStr=single
  Gain5 : Gain  Gain=1.5  ParamDataTypeStr=single
  Product{4..7} (4 alike) : Product
  Selector2 : Selector  InputPortWidth=2  IndexOptions=Index vector (dialog)  Indices=[2 1]  OutputSizes=1
  Selector3 : Selector  InputPortWidth=2  IndexOptions=Index vector (dialog)  Indices=[2 1]  OutputSizes=1
  Sum of Elements3 : Sum  Inputs=+
  P0 : Outport  VectorParamsAs1DForOutWhenUnconnected=off
  Q0 : Outport  Port=2  VectorParamsAs1DForOutWhenUnconnected=off
  wires:
  Demux/2 -> Add/2
  Demux/1 -> Add/1
  Product7/1 -> Add4/2
  Add4/1 -> Sum of Elements3/1
  Product6/1 -> Add4/1
  Sum of Elements3/1 -> Gain5/1
  Gain5/1 -> P0/1
  [IdqP] -> Product6/2
  [VdqP] -> Product6/1
  [IdqN] -> Product7/2
  [VdqN] -> Product7/1
  [VdqN] -> Product5/1
  [IqdN] -> Product5/2
  [VdqP] -> Product4/1
  [IqdP] -> Product4/2
  Selector3/1 -> [IqdN]
  Selector2/1 -> [IqdP]
  Gain4/1 -> Q0/1
  Add/1 -> Gain4/1
  Product4/1 -> Add3/1
  Add3/1 -> Demux/1
  Product5/1 -> Add3/2
  VdqP/1 -> [VdqP]
  IdqzN/1 -> Selector3/1, [IdqN]
  VdqN/1 -> [VdqN]
  IdqzP/1 -> Selector2/1, [IdqP]

== system GCI_Ctrl_PLL_C2000/C2000_SW/CtrlLoop/CurrentController/CurrentControllerAdptv/Subsystem/abc_dqz ==
  abc : Inport
  wtNow : Inport  Port=2
  Subsystem : Subsystem
  Subsystem2 : Subsystem
  dqz : Outport  VectorParamsAs1DForOutWhenUnconnected=off
  wires:
  Subsystem2/1(dq) -> dqz/1
  Subsystem/1(al_be_0) -> Subsystem2/1(alpha_beta)
  abc/1 -> Subsystem/1(abc)
  wtNow/1 -> Subsystem2/2(Ang)

== system GCI_Ctrl_PLL_C2000/C2000_SW/CtrlLoop/CurrentController/CurrentControllerAdptv/Subsystem/dd_dqz1 ==
  abc : Inport
  wtNow : Inport  Port=2
  Delay : Delay  DelayLength=1
  Delay1 : Delay  DelayLength=1
  Gain : Gain  Gain=-1  ParamDataTypeStr=single
  LPF : Subsystem  mask{Ts=1/(Var.PWM_Freq), w=single(2*pi*50), K=single(1), y_0=0}
      mask prompts: Ts "Sample Time (s)"; w "CutOff Freq (-3db) (rad/s)"; K "Gain"; y_0 "Initial output"
  LPF1 : Subsystem  mask{Ts=1/(Var.PWM_Freq), w=single(2*pi*50), K=single(1), y_0=0}
      mask prompts: Ts "Sample Time (s)"; w "CutOff Freq (-3db) (rad/s)"; K "Gain"; y_0 "Initial output"
  Subsystem : Subsystem
  Subsystem1 : Subsystem
  Subsystem2 : Subsystem
  Subsystem3 : Subsystem
  Subsystem4 : Subsystem
  dqzP : Outport  VectorParamsAs1DForOutWhenUnconnected=off
  dqzN : Outport  Port=2  VectorParamsAs1DForOutWhenUnconnected=off
  wires:
  wtNow/1 -> Subsystem4/3(Theta), Subsystem2/2(wtNow), Gain/1
  Subsystem/1(al_be_0) -> Subsystem1/1(alpha_beta), Subsystem2/1(alpha_beta)
  abc/1 -> Subsystem/1(abc)
  Gain/1 -> Subsystem3/3(Theta), Subsystem1/2(wtNow)
  LPF/1(y) -> Delay/1
  LPF1/1(y) -> Delay1/1
  Subsystem3/1(Vdq_out) -> dqzN/1, LPF1/1(u)
  Delay1/1 -> Subsystem4/2(Vdq_Inverse)
  Delay/1 -> Subsystem3/2(Vdq_Inverse)
  Subsystem4/1(Vdq_out) -> dqzP/1, LPF/1(u)
  Subsystem2/1(dq) -> Subsystem4/1(Vdq_in)
  Subsystem1/1(dq) -> Subsystem3/1(Vdq_in)

== system GCI_Ctrl_PLL_C2000/C2000_SW/CtrlLoop/CurrentController/CurrentControllerAdptv/Subsystem/dd_dqz2 ==
  abc : Inport
  wtNow : Inport  Port=2
  Delay : Delay  DelayLength=1
  Delay1 : Delay  DelayLength=1
  Gain : Gain  Gain=-1  ParamDataTypeStr=single
  LPF : Subsystem  mask{Ts=1/(Var.PWM_Freq), w=single(50), K=single(1), y_0=0}
      mask prompts: Ts "Sample Time (s)"; w "CutOff Freq (-3db) (rad/s)"; K "Gain"; y_0 "Initial output"
  LPF1 : Subsystem  mask{Ts=1/(Var.PWM_Freq), w=single(50), K=single(1), y_0=0}
      mask prompts: Ts "Sample Time (s)"; w "CutOff Freq (-3db) (rad/s)"; K "Gain"; y_0 "Initial output"
  Subsystem : Subsystem
  Subsystem1 : Subsystem
  Subsystem2 : Subsystem
  Subsystem3 : Subsystem
  Subsystem4 : Subsystem
  dqzP : Outport  VectorParamsAs1DForOutWhenUnconnected=off
  dqzN : Outport  Port=2  VectorParamsAs1DForOutWhenUnconnected=off
  wires:
  wtNow/1 -> Subsystem2/2(wtNow), Subsystem4/3(Theta), Gain/1
  Subsystem1/1(dq) -> Subsystem3/1(Vdq_in)
  Subsystem2/1(dq) -> Subsystem4/1(Vdq_in)
  Subsystem4/1(Vdq_out) -> dqzP/1, LPF/1(u)
  Delay/1 -> Subsystem3/2(Vdq_Inverse)
  Delay1/1 -> Subsystem4/2(Vdq_Inverse)
  Subsystem3/1(Vdq_out) -> dqzN/1, LPF1/1(u)
  LPF1/1(y) -> Delay1/1
  LPF/1(y) -> Delay/1
  Gain/1 -> Subsystem1/2(wtNow), Subsystem3/3(Theta)
  abc/1 -> Subsystem/1(abc)
  Subsystem/1(al_be_0) -> Subsystem2/1(alpha_beta), Subsystem1/1(alpha_beta)

== system GCI_Ctrl_PLL_C2000/C2000_SW/CtrlLoop/CurrentController/CurrentControllerAdptv/dqz2abc_1/Subsystem ==
  al_be_0 : Inport  OutDataTypeStr=single  PortDimensions=3
  Gain3 : Gain  Gain="single([ 1   0   1; -1/2  sqrt(3)/2   1; -1/2  -sqrt(3)/2  1 ] )"  Multiplication=Matrix(K*u) (u vector)  ParamDataTypeStr=single  OutDataTypeStr=single  SaturateOnIntegerOverflow=on
  abc : Outport  OutDataTypeStr=single  VectorParamsAs1DForOutWhenUnconnected=off
  wires:
  Gain3/1 -> abc/1  "abc"
  al_be_0/1 -> Gain3/1

== system GCI_Ctrl_PLL_C2000/C2000_SW/CtrlLoop/CurrentController/CurrentControllerAdptv/dqz2abc_1/Subsystem1 ==
  note: *
  note: [  cos(wt)   -sin(wt)
      |    sin(wt)    cos(wt)   ]
  note: [  al
      |     be  ]
  note: inv ([  cos(wt)   sin(wt)
      |    -sin(wt)    cos(wt)   ])
  note: [ d
      |    q ]
  note: [  al
      |     be  ]
  note: [ d
      |    q ]
  note: *
  note: =
  note: =
  dqz : Inport  OutDataTypeStr=single  PortDimensions=3
  Ang : Inport  Port=2  OutDataTypeStr=single  PortDimensions=1
  Fcn : Fcn  Expr=u[1]*cos(u[3]) - u[2]*sin(u[3])
  Fcn1 : Fcn  Expr=u[1]*sin(u[3]) + u[2]*cos(u[3])
  Mux1 : Mux  Inputs=3
  Mux2 : Mux  Inputs=[2 1]
  Mux3 : Mux  Inputs=[2 1]
  Selector : Selector  InputPortWidth=3  IndexOptions=Index vector (dialog)  Indices=[1 2]  OutputSizes=1
  Selector1 : Selector  InputPortWidth=3  IndexOptions=Index vector (dialog)  Indices=[3]  OutputSizes=1
  alpha_beta : Outport  OutDataTypeStr=single  InitialOutput=[0,0]  VectorParamsAs1DForOutWhenUnconnected=off
  wires:
  Fcn1/1 -> Mux1/2
  Mux3/1 -> Fcn1/1
  Mux1/1 -> alpha_beta/1
  Mux2/1 -> Fcn/1
  Ang/1 -> Mux2/2, Mux3/2
  Fcn/1 -> Mux1/1
  Selector/1 -> Mux2/1, Mux3/1
  dqz/1 -> Selector1/1, Selector/1
  Selector1/1 -> Mux1/3

== system GCI_Ctrl_PLL_C2000/C2000_SW/CtrlLoop/CurrentController/CurrentControllerAdptv/dqz2abc_2/Subsystem ==
  al_be_0 : Inport  OutDataTypeStr=single  PortDimensions=3
  Gain3 : Gain  Gain="single([ 1   0   1; -1/2  sqrt(3)/2   1; -1/2  -sqrt(3)/2  1 ] )"  Multiplication=Matrix(K*u) (u vector)  ParamDataTypeStr=single  OutDataTypeStr=single  SaturateOnIntegerOverflow=on
  abc : Outport  OutDataTypeStr=single  VectorParamsAs1DForOutWhenUnconnected=off
  wires:
  al_be_0/1 -> Gain3/1
  Gain3/1 -> abc/1

== system GCI_Ctrl_PLL_C2000/C2000_SW/CtrlLoop/CurrentController/CurrentControllerAdptv/dqz2abc_2/Subsystem1 ==
  note: =
  note: =
  note: *
  note: [ d
      |    q ]
  note: [  al
      |     be  ]
  note: [ d
      |    q ]
  note: inv ([  cos(wt)   sin(wt)
      |    -sin(wt)    cos(wt)   ])
  note: [  al
      |     be  ]
  note: [  cos(wt)   -sin(wt)
      |    sin(wt)    cos(wt)   ]
  note: *
  dqz : Inport  OutDataTypeStr=single  PortDimensions=3
  Ang : Inport  Port=2  OutDataTypeStr=single  PortDimensions=1
  Fcn : Fcn  Expr=u[1]*cos(u[3]) - u[2]*sin(u[3])
  Fcn1 : Fcn  Expr=u[1]*sin(u[3]) + u[2]*cos(u[3])
  Mux1 : Mux  Inputs=3
  Mux2 : Mux  Inputs=[2 1]
  Mux3 : Mux  Inputs=[2 1]
  Selector : Selector  InputPortWidth=3  IndexOptions=Index vector (dialog)  Indices=[1 2]  OutputSizes=1
  Selector1 : Selector  InputPortWidth=3  IndexOptions=Index vector (dialog)  Indices=[3]  OutputSizes=1
  alpha_beta : Outport  OutDataTypeStr=single  InitialOutput=[0,0]  VectorParamsAs1DForOutWhenUnconnected=off
  wires:
  Selector1/1 -> Mux1/3
  dqz/1 -> Selector/1, Selector1/1
  Selector/1 -> Mux3/1, Mux2/1
  Fcn/1 -> Mux1/1
  Ang/1 -> Mux3/2, Mux2/2
  Mux2/1 -> Fcn/1
  Mux1/1 -> alpha_beta/1
  Mux3/1 -> Fcn1/1
  Fcn1/1 -> Mux1/2

== system GCI_Ctrl_PLL_C2000/C2000_SW/CtrlLoop/CurrentController/CurrentControllerAdptv2/MESO/CFDL ==
  u_k-1 : Inport
  e_k : Inport  Port=2
  Abs : Abs  SaturateOnIntegerOverflow=off
  Compare To Constant : simulink/Logic and Bit Operations/Compare To Constant  relop=>  const=0  OutDataTypeStr=boolean
  Compare To Constant1 : simulink/Logic and Bit Operations/Compare To Constant  relop=>=  const=ADPTV.k*eye(size(ADPTV.psi0,1),size(ADPTV.psi0,2))  OutDataTypeStr=boolean
  Delta : Gain  Gain=ADPTV.delta
  Divide : Product  Inputs=*/
  Mag : Subsystem
  Product : Product  Multiplication=Matrix(*)
  Product1 : Product  Multiplication=Matrix(*)
  Product3 : Product
  Psi_0 : Constant  Value=ADPTV.psi0
  Reshape : Reshape  OutputDimensionality=Column vector (2-D)
  Square : Math  Operator=square
  Sum : Sum  Inputs=|+-
  Sum1 : Sum  Inputs=|+-
  Sum2 : Sum  Inputs=|+-
  Sum3 : Sum  Inputs=|++
  Sum4 : Sum  Inputs=|++
  Switch : Switch  Criteria=u2 > Threshold  SaturateOnIntegerOverflow=off  InputSameDT=off
  Switch1 : Switch  Criteria=u2 > Threshold  SaturateOnIntegerOverflow=off  InputSameDT=off
  Transpose : Math  Operator=transpose
  Unit Delay : UnitDelay  InitialCondition=ADPTV.psi0  SampleTime=-1  HasFrameUpgradeWarning=on
  Unit Delay1 : UnitDelay  SampleTime=-1  HasFrameUpgradeWarning=on
  Unit Delay2 : UnitDelay  SampleTime=-1  HasFrameUpgradeWarning=on
  eta : Constant  Value=ADPTV.eta
  Phi_k : Outport
  wires:
  Reshape/1 -> Product1/1
  Delta/1 -> Reshape/1
  Switch1/1 -> Unit Delay/1, Phi_k/1
  Compare To Constant1/1 -> Switch1/2
  Abs/1 -> Compare To Constant1/1
  Product3/1 -> Compare To Constant/1
  Switch/1 -> Switch1/1, Abs/1
  Compare To Constant/1 -> Switch/2
  Psi_0/1 -> Product3/2, Switch1/3, Switch/3
  [Phi_k_1] -> Sum4/2
  Divide/1 -> Sum4/1  "$\\frac{\\delta(\\Delta e_{k}-\\hat{\\Phi}_{e,k-1}\\Delta u_{k-1})\\Delta u_{k-1}^T}{\\eta+||\\Delta u_{k-1}||^2}$"
  Square/1 -> Sum3/2  "$||\\Delta u_{k-1}||^2$"
  Sum3/1 -> Divide/2  "$\\eta+||\\Delta u_{k-1}||^2$"
  Product1/1 -> Divide/1  "$\\delta(\\Delta e_{k}-\\hat{\\Phi}_{e,k-1}\\Delta u_{k-1})\\Delta u_{k-1}^T$"
  eta/1 -> Sum3/1
  [Abs_D_u_k_1] -> Square/1
  [D_u_k_1_T] -> Product1/2
  Sum2/1 -> Delta/1
  [D_u_k_1] -> Product/2
  [Phi_k_1] -> Product/1
  Product/1 -> Sum2/2
  [D_e_k] -> Sum2/1
  e_k/1 -> Sum1/1, Unit Delay2/1
  Unit Delay2/1 -> Sum1/2
  Sum1/1 -> [D_e_k]  "$\\Delta e_{k}$"
  Transpose/1 -> [D_u_k_1_T]
  Mag/1(Out1) -> [Abs_D_u_k_1]  "$||\\Delta u_{k-1}||$"
  Sum/1 -> Transpose/1, Mag/1(In1), [D_u_k_1]  "$\\Delta u_{k-1}$"
  Unit Delay1/1 -> Sum/2
  u_k-1/1 -> Unit Delay1/1, Sum/1
  Unit Delay/1 -> [Phi_k_1]  "$\\hat{\\Phi}_{e,k-1}$"
  Sum4/1 -> Switch/1, Product3/1  "Phi_k"

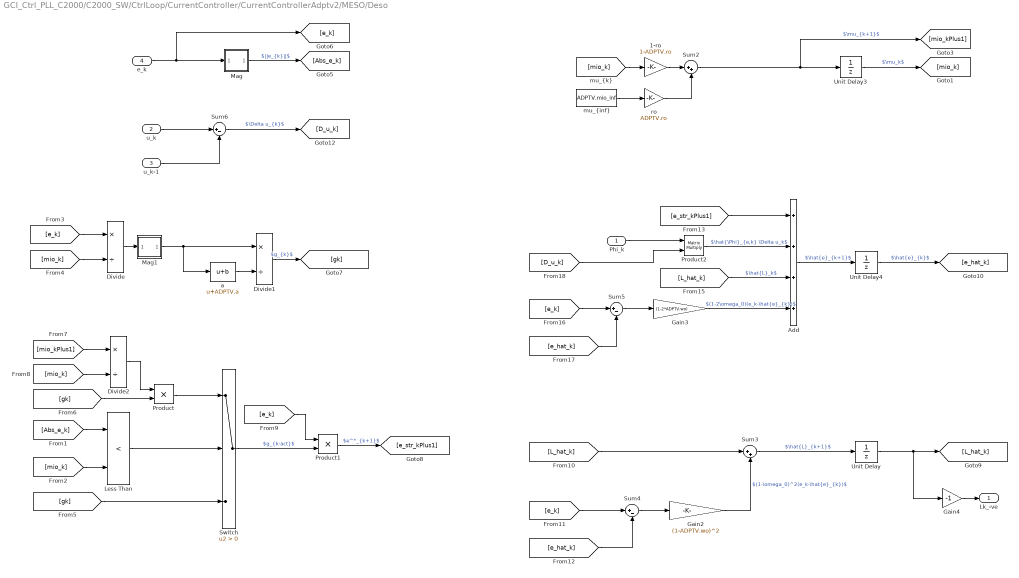
== system GCI_Ctrl_PLL_C2000/C2000_SW/CtrlLoop/CurrentController/CurrentControllerAdptv2/MESO/Deso ==
  Phi_k : Inport
  u_k : Inport  Port=2
  u_k-1 : Inport  Port=3
  e_k : Inport  Port=4
  1-ro : Gain  Gain=1-ADPTV.ro
  Add : Sum  Inputs=++++
  Divide : Product  Inputs=*/
  Divide1 : Product  Inputs=*/
  Divide2 : Product  Inputs=*/
  Gain2 : Gain  Gain=(1-ADPTV.wo)^2
  Gain3 : Gain  Gain=(1-2*ADPTV.wo)
  Gain4 : Gain  Gain=-1
  Less Than : RelationalOperator  Operator=<  OutDataTypeStr=boolean  RndMeth=Simplest  InputSameDT=off
  Mag : Subsystem
  Mag1 : Subsystem
  Product : Product
  Product1 : Product
  Product2 : Product  Multiplication=Matrix(*)
  Sum2 : Sum  Inputs=|++
  Sum3 : Sum  Inputs=|++
  Sum4 : Sum  Inputs=|+-
  Sum5 : Sum  Inputs=|+-
  Sum6 : Sum  Inputs=|+-
  Switch : Switch  Criteria=u2 > Threshold  SaturateOnIntegerOverflow=off  InputSameDT=off
  Unit Delay : UnitDelay  SampleTime=-1  HasFrameUpgradeWarning=on
  Unit Delay3 : UnitDelay  InitialCondition=ADPTV.mio_0  SampleTime=-1  HasFrameUpgradeWarning=on
  Unit Delay4 : UnitDelay  SampleTime=-1  HasFrameUpgradeWarning=on
  a : Bias  Bias=ADPTV.a  SaturateOnIntegerOverflow=off
  "mu_{inf}" : Constant  Value=ADPTV.mio_inf
  ro : Gain  Gain=ADPTV.ro
  Lk_-ve : Outport
  wires:
  u_k-1/1 -> Sum6/2
  Gain3/1 -> Add/4  "$(1-2\\omega_0)(e_k-\\hat{e}_{k})$"
  u_k/1 -> Sum6/1
  Sum6/1 -> [D_u_k]  "$\\Delta u_{k}$"
  Gain4/1 -> Lk_-ve/1
  Sum5/1 -> Gain3/1
  [e_k] -> Sum5/1
  [e_hat_k] -> Sum5/2
  [L_hat_k] -> Add/3  "$\\hat{L}_k$"
  Product2/1 -> Add/2  "$\\hat{\\Phi}_{e,k} \\Delta u_k$"
  [e_str_kPlus1] -> Add/1
  [D_u_k] -> Product2/2
  Phi_k/1 -> Product2/1
  Add/1 -> Unit Delay4/1  "$\\hat{e}_{k+1}$"
  Unit Delay4/1 -> [e_hat_k]  "$\\hat{e}_{k}$"
  Sum3/1 -> Unit Delay/1  "$\\hat{L}_{k+1}$"
  [e_hat_k] -> Sum4/2
  [e_k] -> Sum4/1
  Gain2/1 -> Sum3/2  "$(1-\\omega_0)^2(e_k-\\hat{e}_{k})$"
  Sum4/1 -> Gain2/1
  Unit Delay/1 -> [L_hat_k], Gain4/1
  [L_hat_k] -> Sum3/1
  Product1/1 -> [e_str_kPlus1]  "$e^*_{k+1}$"
  [e_k] -> Product1/1
  Switch/1 -> Product1/2  "$g_{k-act}$"
  Product/1 -> Switch/1
  Divide2/1 -> Product/1
  [gk] -> Product/2
  [mio_kPlus1] -> Divide2/1
  [mio_k] -> Divide2/2
  [gk] -> Switch/3
  Divide1/1 -> [gk]  "$g_{k}$"
  a/1 -> Divide1/2
  Mag1/1(Out1) -> a/1, Divide1/1
  Divide/1 -> Mag1/1(e_k)
  [mio_k] -> Divide/2
  [e_k] -> Divide/1
  Less Than/1 -> Switch/2
  [mio_k] -> Less Than/2
  [Abs_e_k] -> Less Than/1
  Mag/1(Out1) -> [Abs_e_k]  "$||e_{k}||$"
  e_k/1 -> Mag/1(e_k), [e_k]
  [mio_k] -> 1-ro/1
  1-ro/1 -> Sum2/1
  ro/1 -> Sum2/2
  "mu_{inf}"/1 -> ro/1
  Sum2/1 -> Unit Delay3/1, [mio_kPlus1]  "$\\mu_{k+1}$"
  Unit Delay3/1 -> [mio_k]  "$\\mu_k$"

== system GCI_Ctrl_PLL_C2000/C2000_SW/CtrlLoop/CurrentController/CurrentControllerAdptv2/MESO/Lambda ==
  Bias : Bias  Bias=ADPTV.LamdaInf  SaturateOnIntegerOverflow=off
  Constant2 : Constant  Value=ADPTV.Lamda0-ADPTV.LamdaInf
  Constant3 : Constant
  Data Type Conversion : DataTypeConversion  SaturateOnIntegerOverflow=off  RndMeth=Floor
  Discrete-Time Integrator : DiscreteIntegrator  SampleTime=-1  ICPrevOutput=DiscIntNeverNeededParam  ICPrevScaledInput=DiscIntNeverNeededParam
  Gain : Gain  Gain=-ADPTV.b0
  Math Function1 : Math
  Product3 : Product
  $\lambda_k$ : Outport
  wires:
  Data Type Conversion/1 -> Product3/1
  Bias/1 -> $\lambda_k$/1  "$\\lambda_k$"
  Product3/1 -> Bias/1
  Math Function1/1 -> Data Type Conversion/1
  Gain/1 -> Math Function1/1
  Constant3/1 -> Discrete-Time Integrator/1
  Discrete-Time Integrator/1 -> Gain/1
  Constant2/1 -> Product3/2

== system GCI_Ctrl_PLL_C2000/C2000_SW/CtrlLoop/CurrentController/CurrentControllerAdptv2/MESO/Mag ==
  in : Inport
  Reshape : Reshape
  Sqrt : Sqrt
  Square : Math  Operator=square
  Sum of Elements : Sum  Inputs=+
  Abs : Outport
  wires:
  Reshape/1 -> Abs/1
  in/1 -> Square/1
  Square/1 -> Sum of Elements/1
  Sum of Elements/1 -> Sqrt/1
  Sqrt/1 -> Reshape/1
